simulink model "XeCanBangLR"  (R2022b)
settings: Solver=FixedStepAuto  StartTime=0.0  StopTime=50  FixedStep=0.01  RelTol=1e-3
undefined symbols (not defined in the file): Kd, Kd1, Kd2, Ki, Ki1, Ki2, Kp, Kp1, Kp2, x1_init, x2_init, x4_init, x5_init, x7_init, x8_init
settings Model: Creator=Admins  LastModifiedBy=Admins
settings DataIOCC: ReturnWorkspaceOutputs=off

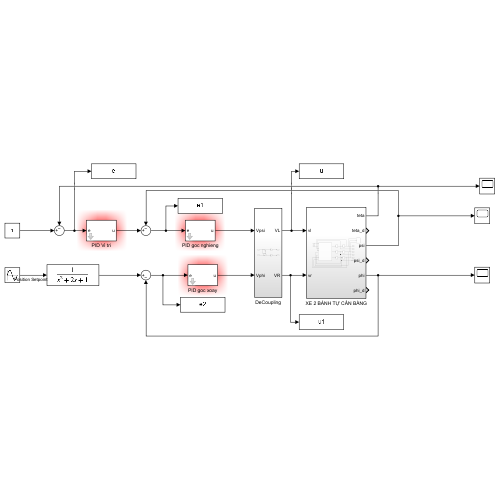
[thumbnail: Simulink's stored preview of the top-level diagram]
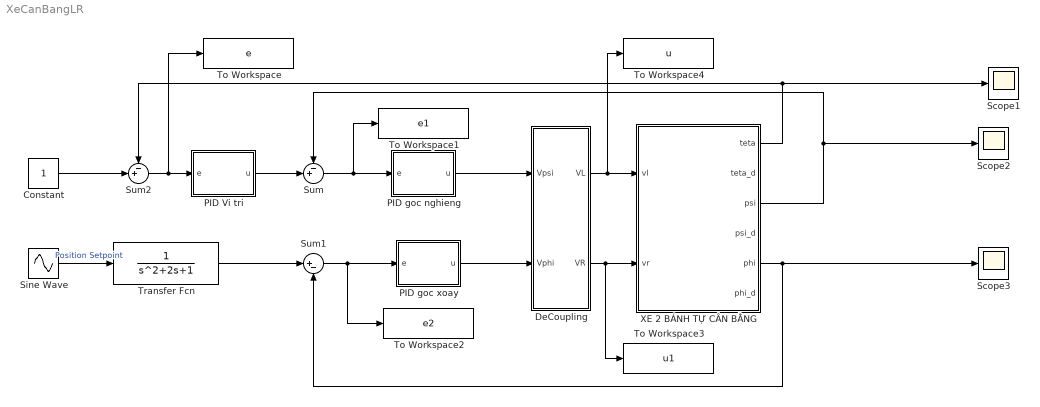
== system XeCanBangLR ==
  Constant : Constant
  DeCoupling : Subsystem
  PID Vi tri : Subsystem  mask{Kp=Kp, Ki=Ki, Kd=Kd, T=0.01}
  PID goc nghieng : Subsystem  mask{Kp=Kp1, Ki=Ki1, Kd=Kd1, T=0.01}
  PID goc xoay : Subsystem  mask{Kp=Kp2, Ki=Ki2, Kd=Kd2, T=0.01}
  Scope1 : Scope
  Scope2 : Scope
  Scope3 : Scope
  Sine Wave : Sin  SampleTime=0
  Sum : Sum  Inputs=-+|
  Sum1 : Sum  Inputs=|+-
  Sum2 : Sum  Inputs=-+|
  To Workspace : ToWorkspace  VariableName=e  SampleTime=-1
  To Workspace1 : ToWorkspace  VariableName=e1  SampleTime=-1
  To Workspace2 : ToWorkspace  VariableName=e2  SampleTime=-1
  To Workspace3 : ToWorkspace  VariableName=u1  SampleTime=-1
  To Workspace4 : ToWorkspace  VariableName=u  SampleTime=-1
  Transfer Fcn : TransferFcn
  XE 2 BÁNH TỰ CÂN BẰNG : Subsystem
  wires:
  DeCoupling/1(VL) -> To Workspace4/1, XE 2 BÁNH TỰ CÂN BẰNG/1(vl)
  DeCoupling/2(VR) -> To Workspace3/1, XE 2 BÁNH TỰ CÂN BẰNG/2(vr)
  PID goc nghieng/1(u) -> DeCoupling/1(Vpsi)
  Sum/1 -> PID goc nghieng/1(e), To Workspace1/1
  PID goc xoay/1(u) -> DeCoupling/2(Vphi)
  Sum1/1 -> PID goc xoay/1(e), To Workspace2/1
  PID Vi tri/1(u) -> Sum/2
  Sum2/1 -> To Workspace/1, PID Vi tri/1(e)
  Transfer Fcn/1 -> Sum1/1
  XE 2 BÁNH TỰ CÂN BẰNG/1(teta) -> Scope1/1, Sum2/1
  XE 2 BÁNH TỰ CÂN BẰNG/3(psi) -> Scope2/1, Sum/1
  XE 2 BÁNH TỰ CÂN BẰNG/5(phi) -> Scope3/1, Sum1/2
  Constant/1 -> Sum2/2
  Sine Wave/1 -> Transfer Fcn/1  "Position Setpoint"

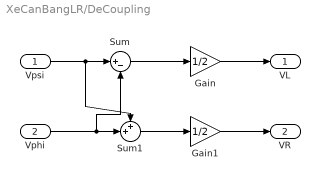
== system XeCanBangLR/DeCoupling ==
  Vpsi : Inport
  Vphi : Inport  Port=2
  Gain : Gain  Gain=1/2
  Gain1 : Gain  Gain=1/2
  Sum : Sum  Inputs=|+-
  Sum1 : Sum  Inputs=++|
  VL : Outport
  VR : Outport  Port=2
  wires:
  Vpsi/1 -> Sum1/1, Sum/1
  Sum/1 -> Gain/1
  Gain/1 -> VL/1
  Vphi/1 -> Sum/2, Sum1/2
  Gain1/1 -> VR/1
  Sum1/1 -> Gain1/1

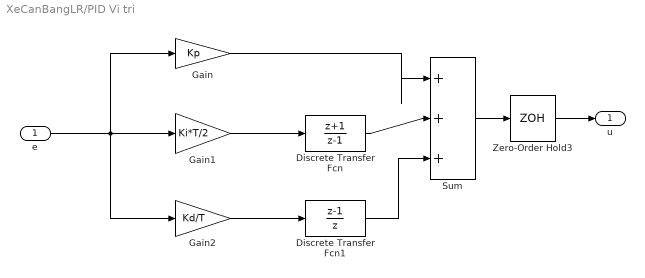
== system XeCanBangLR/PID Vi tri ==
  e : Inport
  Discrete Transfer Fcn : DiscreteTransferFcn  Numerator=[1 1]  Denominator=[1 -1]
  Discrete Transfer Fcn1 : DiscreteTransferFcn  Numerator=[1 -1]  Denominator=[1 0]
  Gain : Gain  Gain=Kp
  Gain1 : Gain  Gain=Ki*T/2
  Gain2 : Gain  Gain=Kd/T
  Sum : Sum  Inputs=|+++
  Zero-Order Hold3 : ZeroOrderHold  SampleTime=0.01
  u : Outport
  wires:
  e/1 -> Gain2/1, Gain1/1, Gain/1
  Gain1/1 -> Discrete Transfer Fcn/1
  Gain2/1 -> Discrete Transfer Fcn1/1
  Discrete Transfer Fcn1/1 -> Sum/3
  Discrete Transfer Fcn/1 -> Sum/2
  Gain/1 -> Sum/1
  Zero-Order Hold3/1 -> u/1
  Sum/1 -> Zero-Order Hold3/1

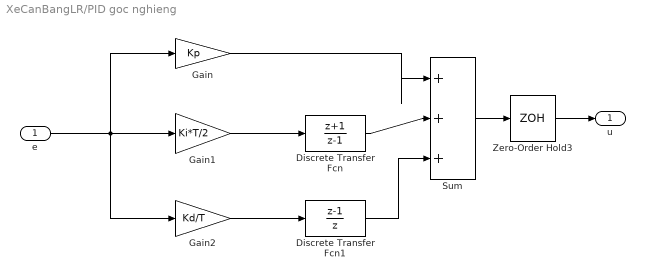
== system XeCanBangLR/PID goc nghieng ==
  e : Inport
  Discrete Transfer Fcn : DiscreteTransferFcn  Numerator=[1 1]  Denominator=[1 -1]
  Discrete Transfer Fcn1 : DiscreteTransferFcn  Numerator=[1 -1]  Denominator=[1 0]
  Gain : Gain  Gain=Kp
  Gain1 : Gain  Gain=Ki*T/2
  Gain2 : Gain  Gain=Kd/T
  Sum : Sum  Inputs=|+++
  Zero-Order Hold3 : ZeroOrderHold  SampleTime=0.01
  u : Outport
  wires:
  Sum/1 -> Zero-Order Hold3/1
  Zero-Order Hold3/1 -> u/1
  Gain/1 -> Sum/1
  Discrete Transfer Fcn/1 -> Sum/2
  Discrete Transfer Fcn1/1 -> Sum/3
  Gain2/1 -> Discrete Transfer Fcn1/1
  Gain1/1 -> Discrete Transfer Fcn/1
  e/1 -> Gain/1, Gain1/1, Gain2/1

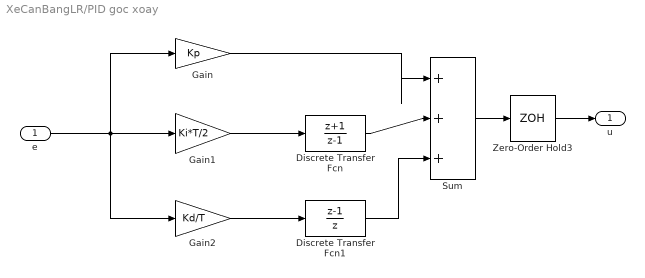
== system XeCanBangLR/PID goc xoay ==
  e : Inport
  Discrete Transfer Fcn : DiscreteTransferFcn  Numerator=[1 1]  Denominator=[1 -1]
  Discrete Transfer Fcn1 : DiscreteTransferFcn  Numerator=[1 -1]  Denominator=[1 0]
  Gain : Gain  Gain=Kp
  Gain1 : Gain  Gain=Ki*T/2
  Gain2 : Gain  Gain=Kd/T
  Sum : Sum  Inputs=|+++
  Zero-Order Hold3 : ZeroOrderHold  SampleTime=0.01
  u : Outport
  wires:
  e/1 -> Gain2/1, Gain1/1, Gain/1
  Gain1/1 -> Discrete Transfer Fcn/1
  Gain2/1 -> Discrete Transfer Fcn1/1
  Discrete Transfer Fcn1/1 -> Sum/3
  Discrete Transfer Fcn/1 -> Sum/2
  Gain/1 -> Sum/1
  Zero-Order Hold3/1 -> u/1
  Sum/1 -> Zero-Order Hold3/1

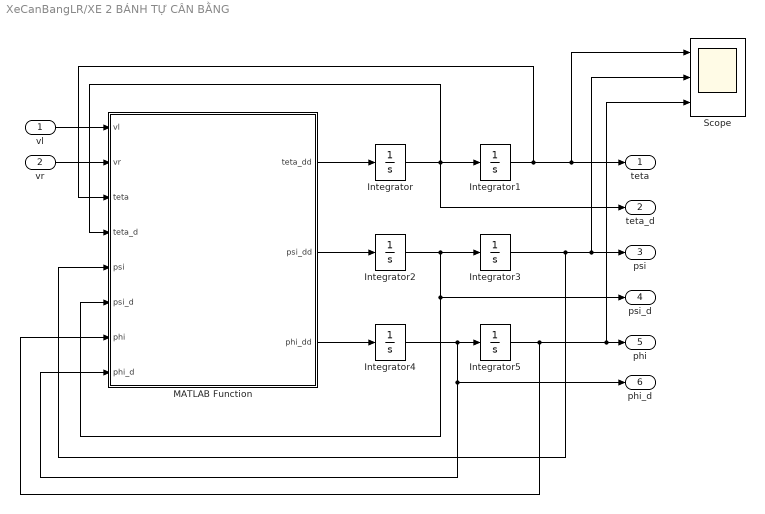
== system XeCanBangLR/XE 2 BÁNH TỰ CÂN BẰNG ==
  vl : Inport
  vr : Inport  Port=2
  Integrator : Integrator  InitialCondition=x2_init
  Integrator1 : Integrator  InitialCondition=x1_init
  Integrator2 : Integrator  InitialCondition=x5_init
  Integrator3 : Integrator  InitialCondition=x4_init
  Integrator4 : Integrator  InitialCondition=x8_init
  Integrator5 : Integrator  InitialCondition=x7_init
  MATLAB Function : MATLAB Function  TreatAsAtomicUnit=on
  Scope : Scope  NumInputPorts=3
  teta : Outport
  teta_d : Outport  Port=2
  psi : Outport  Port=3
  psi_d : Outport  Port=4
  phi : Outport  Port=5
  phi_d : Outport  Port=6
  wires:
  Integrator/1 -> MATLAB Function/4(teta_d), Integrator1/1, teta_d/1
  Integrator1/1 -> MATLAB Function/3(teta), Scope/1, teta/1
  MATLAB Function/1(teta_dd) -> Integrator/1
  Integrator3/1 -> MATLAB Function/5(psi), Scope/2, psi/1
  Integrator2/1 -> MATLAB Function/6(psi_d), psi_d/1, Integrator3/1
  MATLAB Function/2(psi_dd) -> Integrator2/1
  Integrator5/1 -> MATLAB Function/7(phi), Scope/3, phi/1
  Integrator4/1 -> MATLAB Function/8(phi_d), phi_d/1, Integrator5/1
  MATLAB Function/3(phi_dd) -> Integrator4/1
  vl/1 -> MATLAB Function/1(vl)
  vr/1 -> MATLAB Function/2(vr)

== matlab function XeCanBangLR/XE 2 BÁNH TỰ CÂN BẰNG/MATLAB Function ==
  data: vl input; teta_dd output; vr input; teta input; teta_d input; psi input; psi_d input; phi input; phi_d input; psi_dd output; phi_dd output
function [teta_dd,psi_dd,phi_dd] = fcn(vl,vr,teta,teta_d,psi,psi_d,phi,phi_d)

%% Thông số hệ thống xe 2 bánh tự cân bằng dùng LQR
m = 1; %Khoi luong banh xe
M = 5; %Khoi luong robot
R = 0.0725; %ban kinh ban xe
W = 0.24; %Chieu rong robot
D = 0.2; %Chieu sau robot
H = 0.5; %Chieu cao robot
L = 0.18; %khoang cach tu trong tam den truc banh xe
fw = 0.18; %He so ma sat giua banh xe voi mat phang
fm = 0.002; %he so ma sat giua dong co va robot
Jm = 10^-2; %moment quan tinh cua dong co
Jw = m*R^2/2;
J_psi = M*L^2/3;
J_phi = M*(W^2+D^2)/12;
Rm = 50; %Dien tro dong co DC
Kb = 0.468; %he so emf cua dong co
Kt = 0.317; %Momen xoan cua dong co DC
n = 40; %Ty so giam toc
g = 9.81; %Gia toc trong truong
alpha = n*Kt/Rm; beta=n*Kt*Kb/Rm+fm; a =alpha;
T=0.01;

teta_dd = (J_psi*a*vl + J_psi*a*vr - 2*J_psi*beta*teta_d + 2*J_psi*beta*psi_d - 2*J_psi*fw*teta_d + L^2*M*a*vl + L^2*M*a*vr - 2*L^2*M*beta*teta_d + 2*L^2*M*beta*psi_d - 2*L^2*M*fw*teta_d - 4*Jm*fw*n^2*teta_d + L^3*M^2*R*psi_d^2*sin(psi) - 2*L*M*R*beta*teta_d*cos(psi) + 2*L*M*R*beta*psi_d*cos(psi) - L^3*M^2*R*phi_d^2*cos(psi)^2*sin(psi) - L^2*M^2*R*g*cos(psi)*sin(psi) + J_psi*L*M*R*psi_d^2*sin(psi) + 2*Jm*L*M*g*n^2*sin(psi) + L*M*R*a*vl*cos(psi) + L*M*R*a*vr*cos(psi) + 2*Jm*L^2*M*n^2*phi_d^2*cos(psi)*sin(psi) + 2*Jm*L*M*R*n^2*psi_d^2*sin(psi))/(2*J_psi*Jw + L^2*M^2*R^2 + 2*Jw*L^2*M + J_psi*M*R^2 + 2*J_psi*Jm*n^2 + 4*Jm*Jw*n^2 + 2*J_psi*R^2*m + 2*Jm*L^2*M*n^2 + 2*Jm*M*R^2*n^2 + 2*L^2*M*R^2*m + 4*Jm*R^2*m*n^2 - L^2*M^2*R^2*cos(psi)^2 + 4*Jm*L*M*R*n^2*cos(psi));
psi_dd = -(2*Jw*a*vl + 2*Jw*a*vr - 4*Jw*beta*teta_d + 4*Jw*beta*psi_d + M*R^2*a*vl + M*R^2*a*vr - 2*M*R^2*beta*teta_d + 2*M*R^2*beta*psi_d + 2*R^2*a*m*vl + 2*R^2*a*m*vr + 4*Jm*fw*n^2*teta_d - 4*R^2*beta*m*teta_d + 4*R^2*beta*m*psi_d - L*M^2*R^2*g*sin(psi) - 2*Jw*L*M*g*sin(psi) - 2*L*M*R*beta*teta_d*cos(psi) + 2*L*M*R*beta*psi_d*cos(psi) - 2*L*M*R*fw*teta_d*cos(psi) + L^2*M^2*R^2*psi_d^2*cos(psi)*sin(psi) - L^2*M^2*R^2*phi_d^2*cos(psi)*sin(psi) - 2*Jw*L^2*M*phi_d^2*cos(psi)*sin(psi) - 2*Jm*L*M*g*n^2*sin(psi) - 2*L*M*R^2*g*m*sin(psi) + L*M*R*a*vl*cos(psi) + L*M*R*a*vr*cos(psi) - 2*Jm*L^2*M*n^2*phi_d^2*cos(psi)*sin(psi) - 2*L^2*M*R^2*m*phi_d^2*cos(psi)*sin(psi) - 2*Jm*L*M*R*n^2*psi_d^2*sin(psi))/(2*J_psi*Jw + L^2*M^2*R^2 + 2*Jw*L^2*M + J_psi*M*R^2 + 2*J_psi*Jm*n^2 + 4*Jm*Jw*n^2 + 2*J_psi*R^2*m + 2*Jm*L^2*M*n^2 + 2*Jm*M*R^2*n^2 + 2*L^2*M*R^2*m + 4*Jm*R^2*m*n^2 - L^2*M^2*R^2*cos(psi)^2 + 4*Jm*L*M*R*n^2*cos(psi));
phi_dd = -(W^2*beta*phi_d + W^2*fw*phi_d + R*W*a*vl - R*W*a*vr + 4*L^2*M*R^2*psi_d*phi_d*cos(psi)*sin(psi))/(2*J_phi*R^2 + Jm*W^2 + Jm*W^2*n^2 + R^2*W^2*m + 2*L^2*M*R^2*sin(psi)^2);
